simulink model "TargetStatePlant"  (R2019b)
settings: Solver=VariableStepAuto  StartTime=0.0  StopTime=10.0  RelTol=1e-3
undefined symbols (not defined in the file or in its folder): errorMinSpd, heightCalibrating_e, heightDown_e, heightError_e, heightMovingDown_e, heightMovingUp_e, heightUnknown_e, heightUp_e, IOD_OK, IOD_Open, IOD_ScGnd, maxMedianWheelAngle, maxTransitionMachineSpd, minTransitionMachineSpd, trackWidthMax, trackWidthMin, trackWidthTolerance, twoWheelSteer
settings Model: Creator=lemaya  LastModifiedBy=lemaya

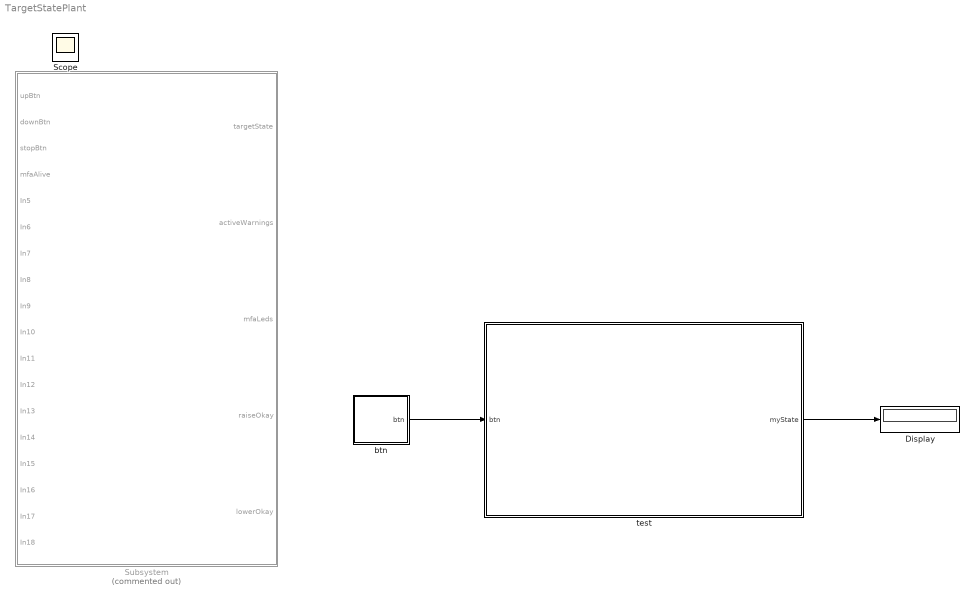
== system TargetStatePlant ==
  Display : Display
  Subsystem : Subsystem  Commented=on
  btn : Stateflow chart  BlockKeywords=__PRM__SERIALIZED__DATA__:Stateflow Chart,Stateflow Diagram  TreatAsAtomicUnit=on
  test : Stateflow chart  BlockKeywords=__PRM__SERIALIZED__DATA__:Stateflow Chart,Stateflow Diagram  TreatAsAtomicUnit=on
  Scope : Scope
  wires:
  test/1(myState) -> Display/1
  btn/1(btn) -> test/1(btn)

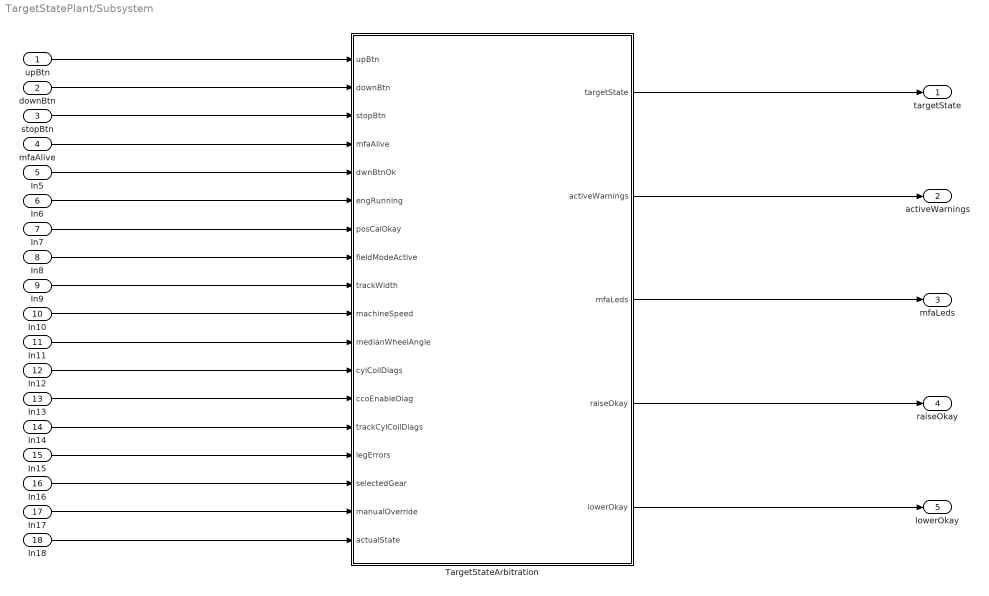
== system TargetStatePlant/Subsystem ==
  upBtn : Inport
  downBtn : Inport  Port=2
  stopBtn : Inport  Port=3
  mfaAlive : Inport  Port=4
  In5 : Inport  Port=5
  In6 : Inport  Port=6
  In7 : Inport  Port=7
  In8 : Inport  Port=8
  In9 : Inport  Port=9
  In10 : Inport  Port=10
  In11 : Inport  Port=11
  In12 : Inport  Port=12
  In13 : Inport  Port=13
  In14 : Inport  Port=14
  In15 : Inport  Port=15
  In16 : Inport  Port=16
  In17 : Inport  Port=17
  In18 : Inport  Port=18
  TargetStateArbitration : Stateflow chart  TreatAsAtomicUnit=on
  targetState : Outport
  activeWarnings : Outport  Port=2
  mfaLeds : Outport  Port=3
  raiseOkay : Outport  Port=4
  lowerOkay : Outport  Port=5
  wires:
  TargetStateArbitration/2(activeWarnings) -> activeWarnings/1
  In8/1 -> TargetStateArbitration/8(fieldModeActive)
  In5/1 -> TargetStateArbitration/5(dwnBtnOk)
  TargetStateArbitration/5(lowerOkay) -> lowerOkay/1
  In16/1 -> TargetStateArbitration/16(selectedGear)
  In18/1 -> TargetStateArbitration/18(actualState)
  TargetStateArbitration/4(raiseOkay) -> raiseOkay/1
  In17/1 -> TargetStateArbitration/17(manualOverride)
  upBtn/1 -> TargetStateArbitration/1(upBtn)
  downBtn/1 -> TargetStateArbitration/2(downBtn)
  In7/1 -> TargetStateArbitration/7(posCalOkay)
  In15/1 -> TargetStateArbitration/15(legErrors)
  TargetStateArbitration/1(targetState) -> targetState/1
  In14/1 -> TargetStateArbitration/14(trackCylCoilDiags)
  In6/1 -> TargetStateArbitration/6(engRunning)
  In11/1 -> TargetStateArbitration/11(medianWheelAngle)
  In12/1 -> TargetStateArbitration/12(cylCoilDiags)
  In13/1 -> TargetStateArbitration/13(ccoEnableDiag)
  In9/1 -> TargetStateArbitration/9(trackWidth)
  In10/1 -> TargetStateArbitration/10(machineSpeed)
  TargetStateArbitration/3(mfaLeds) -> mfaLeds/1
  stopBtn/1 -> TargetStateArbitration/3(stopBtn)
  mfaAlive/1 -> TargetStateArbitration/4(mfaAlive)

== stateflow chart TargetStatePlant/btn ==
  state Off
    en: btn = 0;
  state On
    en: btn = 1;
  (default) -> Off
  Off -> On : after(2,sec)
  On -> Off : after(1,sec)
  data: btn output boolean

== stateflow chart TargetStatePlant/test ==
  state state1
    en: myState = 1;
  state state2
    en: myState = 2;
  state b = leaveState [function]
    (default) -> (junction 8)
    (junction 8) -> (junction 11) [order 1] : [hasChangedTo(btn,1)]
    (junction 11) -> (junction 12) : [myState == 1]
    (junction 8) -> (junction 17) [order 2]
    (junction 12) -> (junction 15) : {b = 1}
    (junction 17) -> (junction 15) : {b = 0}
  (default) -> state1
  state1 -> state2 : [leaveState()]
  state2 -> state1 : [leaveState()]
  data: b function_output double; myState output uint8; btn input boolean

== stateflow chart TargetStatePlant/Subsystem/TargetStateArbitration ==
  state states
    en,du: lowerOkay = ( okayToLower() && !disableLower() );
    raiseOkay = ( okayToRaise() && !disableRiase() );
    state b = leaveActiveState [function]
      (default) -> (junction 1676)
      (junction 1676) -> (junction 1685) [order 1] : [hasChangedTo(stopBtn,1)]
      (junction 1685) -> (junction 1686) [order 1] : [prevTargetState == heightDown_e]
      (junction 1676) -> (junction 1696) [order 2]
      (junction 1685) -> (junction 1687) [order 2]
      (junction 1686) -> (junction 1690)
      (junction 1687) -> (junction 1690) : [prevTargetState == heightUp_e]
      (junction 1690) -> (junction 1698)
      (junction 1696) -> (junction 1698) [order 1] : [manualOverride != 0]
      (junction 1696) -> (junction 1701) [order 2]
      (junction 1698) -> (junction 1700)
      (junction 1701) -> (junction 1700) [order 1] : [!calOkay()]
      (junction 1701) -> (junction 1711) [order 2]
      (junction 1700) -> (junction 1712)
      (junction 1711) -> (junction 1705) [order 1] : [prevTargetState == heightMovingDown_e]
      (junction 1705) -> (junction 1712) : [disableLower()]
      (junction 1711) -> (junction 1713) [order 2]
      (junction 1712) -> (junction 1714)
      (junction 1713) -> (junction 1706) [order 1] : [prevTargetState == heightMovingUp_e]
      (junction 1706) -> (junction 1714) : [disableRiase()]
      (junction 1713) -> (junction 1716) [order 2]
      (junction 1714) -> (junction 1717)
      (junction 1716) -> (junction 1717) [order 1] : [noMovementErr()]
      (junction 1716) -> (junction 1742) [order 2]
      (junction 1717) -> (junction 1734)
      (junction 1742) -> (junction 1733) [order 2] : [hasChangedTo(downBtn,1)]
      (junction 1733) -> (junction 1734) : [prevTargetState == heightMovingDown_e]
      (junction 1742) -> (junction 1744) [order 1]
      (junction 1734) -> (junction 1738)
      (junction 1744) -> (junction 1737) [order 1] : [hasChangedTo(downBtn,1)]
      (junction 1737) -> (junction 1738) : [prevTargetState == heightMovingUp_e]
      (junction 1744) -> (junction 1725) [order 2]
      (junction 1738) -> (junction 1728)
      (junction 1728) -> (junction 1730) : {b = true}
      (junction 1730) -> (junction 1723)
      (junction 1725) -> (junction 1723) : {b = false}
    state clearWarnings [function]
      (default) -> (junction 687) : {activeWarnings.trackWidth = 0;
          | activeWarnings.speed = 0;
          | activeWarnings.guide = 0;
          | activeWarnings.was = 0;
          | activeWarnings.fws = 0;
          | activeWarnings.fieldRoad = 0;
          | activeWarnings.cal = 0;
          | activeWarnings.parkBrake = 0;}
    state upWarnings [function]
      (default) -> (junction 973) : {activeWarnings.trackWidth = !trackWidthOkay();
          | activeWarnings.speed = !speedOkay();
          | activeWarnings.guide = 0;
          | activeWarnings.was = !wasOkay();
          | activeWarnings.fws = 0;
          | activeWarnings.fieldRoad = !fieldModeActive;
          | activeWarnings.cal = !calOkay();
          | activeWarnings.parkBrake = 0;}
    state downWarnings [function]
      (default) -> (junction 976) : {activeWarnings.trackWidth = !trackWidthOkay();
          | activeWarnings.speed = !speedOkay();
          | activeWarnings.guide = 0;
          | activeWarnings.was = !wasOkay();
          | activeWarnings.fws = 0;
          | activeWarnings.fieldRoad = !fieldModeActive;
          | activeWarnings.cal = !calOkay();
          | activeWarnings.parkBrake = !parkBrakeOkay();}
    state doNothing
      en:
      targetState = heightUnknown_e;
      clearWarnings();
      mfaLeds.downBtn = 0;
      mfaLeds.upBtn = 0;
    state active
      en: clearWarnings();
      (history)
      state paused
        en:
        targetState = heightUnknown_e;
      state wait
        en:
        clearWarnings();
      state out = pauseTransition [function]
        (default) -> (junction 927)
        (junction 927) -> (junction 981) [order 1] : [targetState == heightMovingUp_e]
        (junction 981) -> (junction 931) : [!okayToRaise()]
        (junction 931) -> (junction 984) : {upWarnings()}
        (junction 927) -> (junction 933) [order 2]
        (junction 984) -> (junction 937)
        (junction 986) -> (junction 988) : [!okayToLower()]
        (junction 988) -> (junction 937) : {downWarnings()}
        (junction 933) -> (junction 986) [order 1] : [targetState == heightMovingDown_e]
        (junction 933) -> (junction 991) [order 2]
        (junction 937) -> (junction 938) : {out = true}
        (junction 991) -> (junction 932)
        (junction 932) -> (junction 938) : {out = false}
      state out = restartTransition [function]
        (default) -> (junction 1027)
        (junction 1027) -> (junction 1028) [order 1] : [prevTargetState == heightMovingUp_e]
        (junction 1028) -> (junction 1029) : [okayToRaise()]
        (junction 1027) -> (junction 1030) [order 2]
        (junction 1029) -> (junction 1032)
        (junction 1030) -> (junction 1031) [order 1] : [prevTargetState == heightMovingDown_e]
        (junction 1031) -> (junction 1032) : [okayToLower()]
        (junction 1030) -> (junction 1034) [order 2]
        (junction 1032) -> (junction 1035) : {out = true}
        (junction 1034) -> (junction 1035) : {out = false}
      state transitioning
        (history)
        state up
          en:
          targetState = heightMovingUp_e;
          prevTargetState = heightMovingUp_e;
          mfaLeds.upBtn = 2;
          mfaLeds.downBtn = 0;
        state down
          en:
          targetState = heightMovingDown_e;
          prevTargetState = heightMovingDown_e;
          mfaLeds.upBtn = 0;
          mfaLeds.downBtn = 2;
      state holdUp
        en:
        targetState = heightUp_e;
        prevTargetState = heightUp_e;
        mfaLeds.upBtn = 1;
        mfaLeds.downBtn = 0;
      state holdDown
        en:
        targetState = heightDown_e;
        prevTargetState = heightDown_e;
        mfaLeds.upBtn = 0;
        mfaLeds.downBtn = 1;
      paused -> wait : after(20,msec)
      transitioning -> paused : [pauseTransition()]
      wait -> (junction 1563) : [restartTransition()]
      (junction 1563) -> transitioning
      up -> holdUp : [actualState == heightUp_e]
      down -> holdDown : [actualState == heightDown_e]
    state updateWarningsUp
      en: upWarnings();
    state updateWarningsDown
      en: downWarnings();
    state waitForEngineRunning
      en:
      targetState = heightUnknown_e;
      mfaLeds.downBtn = 0;
      mfaLeds.upBtn = 0;
    state out = okayToLower [function]
      (junction 1653) -> (junction 1652) : [trackWidthOkay()]
      (junction 741) -> (junction 1653) [order 2]
      (junction 1652) -> (junction 742)
      (default) -> (junction 737)
      (junction 739) -> (junction 740)
      (junction 737) -> (junction 1545) [order 1] : [parkBrakeOkay()]
      (junction 1545) -> (junction 738) : [speedOkay()]
      (junction 738) -> (junction 739) : [wasOkay()]
      (junction 740) -> (junction 741) : [fieldModeActive]
      (junction 741) -> (junction 742) [order 1] : [trackWidthError()]
      (junction 737) -> (junction 743) [order 2]
      (junction 742) -> (junction 748) : {out = true}
      (junction 743) -> (junction 748) : {out = false}
    state out = disableLower [function]
      (default) -> (junction 1251)
      (junction 1251) -> (junction 1400) [order 1] : [prevTargetState == heightMovingDown_e]
      (junction 1400) -> (junction 1252) : [!mfaAlive]
      (junction 1251) -> (junction 1415) [order 2]
      (junction 1252) -> (junction 1407)
      (junction 1415) -> (junction 1265)
      (junction 1407) -> (junction 1266) : {out = true}
      (junction 1265) -> (junction 1266) : {out = false}
    state out = trackWidthError [function]
      (default) -> (junction 834)
      (junction 834) -> (junction 835) [order 1] : [trackWidth.FrontLeft <= 0]
      (junction 834) -> (junction 836) [order 2]
      (junction 835) -> (junction 837)
      (junction 836) -> (junction 837) [order 1] : [trackWidth.FrontRight <= 0]
      (junction 836) -> (junction 838) [order 2]
      (junction 837) -> (junction 839)
      (junction 838) -> (junction 839) [order 1] : [trackWidth.RearLeft <= 0]
      (junction 838) -> (junction 840) [order 2]
      (junction 839) -> (junction 841)
      (junction 840) -> (junction 841) [order 1] : [trackWidth.RearRight <= 0]
      (junction 840) -> (junction 842) [order 2] : {out = false}
      (junction 841) -> (junction 843) : {out = true}
      (junction 843) -> (junction 842)
    state out = trackRngCheck(width) [function]
      (default) -> (junction 782)
      (junction 782) -> (junction 783) [order 1] : [!trackWidthError()]
      (junction 783) -> (junction 784) : [width >= (trackWidthMin - trackWidthTolerance)]
      (junction 782) -> (junction 785) [order 2] : {out = false}
      (junction 784) -> (junction 786) : [width <= (trackWidthMax + trackWidthTolerance)]
      (junction 786) -> (junction 785) : {out = true}
    state out = requireSpeed [function]
      (default) -> (junction 718)
      (junction 718) -> (junction 719) [commented out] : [trackWidthError()]
      (junction 719) -> (junction 721) [commented out]
      (junction 718) -> (junction 720)
      (junction 720) -> (junction 721) [commented out] : [actualState == heightError_e]
      (junction 720) -> (junction 1581)
      (junction 721) -> (junction 1579) [commented out]
      (junction 1581) -> (junction 1579) [commented out] : [!calOkay()]
      (junction 1581) -> (junction 1107)
      (junction 1579) -> (junction 1109) [commented out]
      (junction 1107) -> (junction 1109) [commented out] : [(cylCoilDiags.retract.FrontLeft & IOD_Open) == IOD_Open]
      (junction 1107) -> (junction 1113)
      (junction 1109) -> (junction 1114) [commented out]
      (junction 1113) -> (junction 1114) [commented out] : [(cylCoilDiags.retract.FrontRight & IOD_Open) == IOD_Open]
      (junction 1114) -> (junction 1122) [commented out]
      (junction 1113) -> (junction 1121)
      (junction 1121) -> (junction 1122) [commented out] : [(cylCoilDiags.retract.RearLeft & IOD_Open) == IOD_Open]
      (junction 1122) -> (junction 1125) [commented out]
      (junction 1121) -> (junction 1124)
      (junction 1124) -> (junction 1125) [commented out] : [(cylCoilDiags.retract.RearRight & IOD_Open) == IOD_Open]
      (junction 1125) -> (junction 722) [commented out]
      (junction 1124) -> (junction 1180)
      (junction 1180) -> (junction 722) [commented out] : [trackCylError()]
      (junction 1180) -> (junction 723)
      (junction 722) -> (junction 724) [commented out] : {out = true}
      (junction 723) -> (junction 724) : {out = false}
    state out = calOkay [function]
      (default) -> (junction 768)
      (junction 768) -> (junction 769) [order 1] : [actualState != heightCalibrating_e]
      (junction 768) -> (junction 771) [order 2] : {out = false}
      (junction 769) -> (junction 770) : [posCalOkay]
      (junction 770) -> (junction 772) : {out = true}
      (junction 771) -> (junction 772)
    state out = wasOkay [function]
      note: %No Front wheel angle requirement
      (default) -> (junction 795)
      (junction 795) -> (junction 1667) [order 1] : [1==1]
      (junction 795) -> (junction 1663) [order 2] : [abs(medianWheelAngle) > maxMedianWheelAngle]
      (junction 1667) -> (junction 1668)
      (junction 795) -> (junction 1665) [order 3] : [!prevWasOkayOut]
      (junction 1663) -> (junction 798) : {out = false}
      (junction 1665) -> (junction 796) : [abs(medianWheelAngle) <= (maxMedianWheelAngle - 2)]
      (junction 1668) -> (junction 796)
      (junction 796) -> (junction 798) : {out = true}
      (junction 798) -> (junction 1660) : {prevWasOkayOut = out}
    state out = targetStateSelected [function]
      (default) -> (junction 1068)
      (junction 1068) -> (junction 1069) [order 1] : [targetState == heightDown_e]
      (junction 1068) -> (junction 1070) [order 2]
      (junction 1069) -> (junction 1071)
      (junction 1070) -> (junction 1071) [order 1] : [targetState == heightUp_e]
      (junction 1070) -> (junction 1085) [order 2]
      (junction 1071) -> (junction 1091)
      (junction 1085) -> (junction 1091) [order 1] : [targetState == heightMovingUp_e]
      (junction 1085) -> (junction 1092) [order 2]
      (junction 1091) -> (junction 1087)
      (junction 1092) -> (junction 1087) [order 1] : [targetState == heightMovingDown_e]
      (junction 1092) -> (junction 1073) [order 2]
      (junction 1087) -> (junction 1074) : {out = true}
      (junction 1073) -> (junction 1074) : {out = false}
    state out = okayToRaise [function]
      (default) -> (junction 894)
      (junction 1304) -> (junction 1298)
      (junction 894) -> (junction 1547) [order 1]
      (junction 1547) -> (junction 1247)
      (junction 1247) -> (junction 1195) : [trackWidthOkay()]
      (junction 1195) -> (junction 1305) : [speedOkay()]
      (junction 1305) -> (junction 1304) : [wasOkay()]
      (junction 1298) -> (junction 896) : [fieldModeActive]
      (junction 894) -> (junction 897) [order 2]
      (junction 896) -> (junction 899) : {out = true}
      (junction 897) -> (junction 899) : {out = false}
    state out = disableRiase [function]
      (default) -> (junction 1420)
      (junction 1420) -> (junction 1448) [order 1] : [prevTargetState == heightMovingUp_e]
      (junction 1448) -> (junction 1635) [order 1] : [!mfaAlive]
      (junction 1420) -> (junction 1423) [order 2]
      (junction 1448) -> (junction 1421) [order 2]
      (junction 1635) -> (junction 1422)
      (junction 1423) -> (junction 1421) [order 1] : [prevTargetState == heightDown_e]
      (junction 1421) -> (junction 1422) [order 1] : [trackWidthError()]
      (junction 1423) -> (junction 1426) [order 2]
      (junction 1421) -> (junction 1424) [order 2]
      (junction 1422) -> (junction 1425)
      (junction 1424) -> (junction 1425) [order 1] : [trackCylError()]
      (junction 1424) -> (junction 1647) [order 2]
      (junction 1425) -> (junction 1650)
      (junction 1647) -> (junction 1650) [order 1] : [!dwnBtnOk]
      (junction 1647) -> (junction 1457) [order 2]
      (junction 1650) -> (junction 1446)
      (junction 1457) -> (junction 1446) [order 1] : [actualState == heightError_e]
      (junction 1457) -> (junction 1464) [order 2]
      (junction 1446) -> (junction 1466)
      (junction 1464) -> (junction 1466) [order 1] : [cylCoilDiags.extend.FrontLeft != IOD_OK]
      (junction 1464) -> (junction 1470) [order 2]
      (junction 1466) -> (junction 1468)
      (junction 1470) -> (junction 1468) [order 1] : [cylCoilDiags.extend.FrontRight != IOD_OK]
      (junction 1470) -> (junction 1473) [order 2]
      (junction 1468) -> (junction 1471)
      (junction 1473) -> (junction 1471) [order 1] : [cylCoilDiags.extend.RearLeft != IOD_OK]
      (junction 1473) -> (junction 1476) [order 2]
      (junction 1471) -> (junction 1474)
      (junction 1476) -> (junction 1474) [order 1] : [cylCoilDiags.extend.RearRight != IOD_OK]
      (junction 1476) -> (junction 1495) [order 2]
      (junction 1474) -> (junction 1485)
      (junction 1495) -> (junction 1485) [order 1] : [cylCoilDiags.retract.FrontLeft != IOD_OK]
      (junction 1495) -> (junction 1489) [order 2]
      (junction 1485) -> (junction 1487)
      (junction 1489) -> (junction 1487) [order 1] : [cylCoilDiags.retract.FrontRight != IOD_OK]
      (junction 1489) -> (junction 1488) [order 2]
      (junction 1487) -> (junction 1484)
      (junction 1488) -> (junction 1484) [order 1] : [cylCoilDiags.retract.RearLeft != IOD_OK]
      (junction 1488) -> (junction 1498) [order 2]
      (junction 1484) -> (junction 1493)
      (junction 1498) -> (junction 1493) [order 1] : [cylCoilDiags.retract.RearRight != IOD_OK]
      (junction 1498) -> (junction 1452) [order 2]
      (junction 1493) -> (junction 1427) : {out = true}
      (junction 1426) -> (junction 1452)
      (junction 1452) -> (junction 1427) : {out = false}
    state out = trackCylError [function]
      (default) -> (junction 1136)
      (junction 1136) -> (junction 1137) [order 1] : [trackCylCoilDiags.extend.FrontLeft != IOD_OK]
      (junction 1136) -> (junction 1138) [order 2]
      (junction 1137) -> (junction 1139)
      (junction 1138) -> (junction 1139) [order 1] : [trackCylCoilDiags.extend.FrontRight != IOD_OK]
      (junction 1138) -> (junction 1140) [order 2]
      (junction 1139) -> (junction 1141)
      (junction 1140) -> (junction 1141) [order 1] : [trackCylCoilDiags.extend.RearLeft != IOD_OK]
      (junction 1140) -> (junction 1142) [order 2]
      (junction 1141) -> (junction 1143)
      (junction 1142) -> (junction 1143) [order 1] : [trackCylCoilDiags.extend.RearRight != IOD_OK]
      (junction 1142) -> (junction 1163) [order 2]
      (junction 1143) -> (junction 1167)
      (junction 1163) -> (junction 1167) [order 1] : [trackCylCoilDiags.retract.FrontLeft != IOD_OK]
      (junction 1163) -> (junction 1161) [order 2]
      (junction 1167) -> (junction 1160)
      (junction 1161) -> (junction 1160) [order 1] : [trackCylCoilDiags.retract.FrontRight != IOD_OK]
      (junction 1161) -> (junction 1162) [order 2]
      (junction 1160) -> (junction 1170)
      (junction 1162) -> (junction 1170) [order 1] : [trackCylCoilDiags.retract.RearLeft != IOD_OK]
      (junction 1162) -> (junction 1174) [order 2]
      (junction 1170) -> (junction 1173)
      (junction 1174) -> (junction 1173) [order 1] : [trackCylCoilDiags.retract.RearRight != IOD_OK]
      (junction 1174) -> (junction 1144) [order 2] : {out = false}
      (junction 1173) -> (junction 1145) : {out = true}
      (junction 1145) -> (junction 1144)
    state out = trackWidthOkay [function]
      (default) -> (junction 807)
      (junction 807) -> (junction 806) [order 2]
      (junction 806) -> (junction 808)
      (junction 807) -> (junction 809) [order 1] : [trackRngCheck(trackWidth.FrontLeft)]
      (junction 809) -> (junction 808) [order 2]
      (junction 808) -> (junction 810)
      (junction 809) -> (junction 811) [order 1] : [trackRngCheck(trackWidth.FrontRight)]
      (junction 811) -> (junction 810) [order 2]
      (junction 810) -> (junction 812)
      (junction 811) -> (junction 813) [order 1] : [trackRngCheck(trackWidth.RearLeft)]
      (junction 813) -> (junction 812) [order 2]
      (junction 812) -> (junction 815) : {out = false}
      (junction 813) -> (junction 814) [order 1] : [trackRngCheck(trackWidth.RearRight)]
      (junction 814) -> (junction 816) : {out = true}
      (junction 815) -> (junction 816)
    state out = speedOkay [function]
      (default) -> (junction 871)
      (junction 871) -> (junction 872) [order 1] : [requireSpeed()]
      (junction 872) -> (junction 873) : [machineSpeed > errorMinSpd]
      (junction 871) -> (junction 874) [order 2]
      (junction 873) -> (junction 875)
      (junction 874) -> (junction 875) [order 1] : [machineSpeed >= minTransitionMachineSpd]
      (junction 875) -> (junction 876) [order 1] : [machineSpeed <= maxTransitionMachineSpd]
      (junction 874) -> (junction 879) [order 2]
      (junction 875) -> (junction 877) [order 2]
      (junction 876) -> (junction 878) : {out = true}
      (junction 877) -> (junction 878) : {out = false}
      (junction 879) -> (junction 877)
    state out = targetStateDown [function]
      (default) -> (junction 1320)
      (junction 1320) -> (junction 1321) [order 1] : [targetState == heightDown_e]
      (junction 1320) -> (junction 1322) [order 2]
      (junction 1321) -> (junction 1323)
      (junction 1322) -> (junction 1323) [order 1] : [targetState == heightMovingDown_e]
      (junction 1322) -> (junction 1334) [order 2]
      (junction 1323) -> (junction 1335) : {out = true}
      (junction 1334) -> (junction 1335) : {out = false}
    state out = targetStateUp [function]
      (default) -> (junction 1361)
      (junction 1361) -> (junction 1362) [order 1] : [targetState == heightUp_e]
      (junction 1361) -> (junction 1363) [order 2]
      (junction 1362) -> (junction 1364)
      (junction 1363) -> (junction 1364) [order 1] : [targetState == heightMovingUp_e]
      (junction 1363) -> (junction 1375) [order 2]
      (junction 1364) -> (junction 1376) : {out = true}
      (junction 1375) -> (junction 1376) : {out = false}
    state out = noMovementErr [function]
      (default) -> (junction 1516)
      (junction 1516) -> (junction 1518) [order 1] : [legErrors.FrontLeft.noMovementErr]
      (junction 1516) -> (junction 1515) [order 2]
      (junction 1518) -> (junction 1520)
      (junction 1515) -> (junction 1520) [order 1] : [legErrors.FrontRight.noMovementErr]
      (junction 1515) -> (junction 1517) [order 2]
      (junction 1520) -> (junction 1522)
      (junction 1517) -> (junction 1522) [order 1] : [legErrors.RearLeft.noMovementErr]
      (junction 1517) -> (junction 1519) [order 2]
      (junction 1522) -> (junction 1523)
      (junction 1519) -> (junction 1523) [order 1] : [legErrors.RearRight.noMovementErr]
      (junction 1519) -> (junction 1524) [order 2] : {out = false}
      (junction 1523) -> (junction 1525) : {out = true}
      (junction 1524) -> (junction 1525)
    state out = parkBrakeOkay [function]
      (default) -> (junction 1551)
      (junction 1551) -> (junction 1552) [order 1] : [selectedGear != 251]
      (junction 1551) -> (junction 1553) [order 2] : {out = false}
      (junction 1552) -> (junction 1554) : {out = true}
      (junction 1554) -> (junction 1553)
    active -> doNothing [order 1] : [leaveActiveState()]
    (junction 705) -> doNothing [order 2]
    (junction 705) -> active [order 1] : [targetStateSelected()]
    updateWarningsUp -> (junction 705) : after(20,msec)
    (junction 1628) -> up : [!disableRiase()]
    (junction 1624) -> (junction 1628) [order 2] : [okayToRaise()]
    (junction 1569) -> holdUp
    (junction 1567) -> (junction 1569)
    (junction 267) -> updateWarningsUp [order 2]
    doNothing -> (junction 267) [order 1] : [hasChangedTo(upBtn,1)]
    (junction 267) -> (junction 1624) [order 1] : [calOkay()]
    (junction 1624) -> holdUp [order 1] : [actualState == heightUp_e]
    (junction 270) -> (junction 267)
    (junction 1197) -> (junction 270) : [targetStateDown()]
    active -> (junction 1197) [order 2] : [hasChangedTo(upBtn,1)]
    (junction 1199) -> (junction 282) : [targetStateUp()]
    active -> (junction 1199) [order 3] : [hasChangedTo(downBtn,1)]
    (junction 282) -> (junction 125)
    doNothing -> (junction 125) [order 2] : [hasChangedTo(downBtn,1)]
    (junction 125) -> (junction 1619) [order 1] : [calOkay()]
    (junction 1619) -> holdDown [order 1] : [actualState == heightDown_e]
    (junction 125) -> updateWarningsDown [order 2]
    (junction 1619) -> (junction 1630) [order 2] : [okayToLower() ]
    (junction 1630) -> down : [!disableLower()]
    updateWarningsDown -> (junction 702) : after(20,msec)
    (junction 1566) -> holdDown [order 1] : [actualState == heightDown_e]
    (junction 702) -> doNothing [order 2]
    (junction 702) -> active [order 1] : [targetStateSelected()]
    (junction 1575) -> doNothing
    (junction 1613) -> (junction 1575)
    (junction 1616) -> (junction 1613)
    (junction 1566) -> (junction 1616) [order 2]
    (junction 1609) -> (junction 1613) [order 2]
    (junction 1611) -> (junction 1616) [order 2]
    (junction 1572) -> (junction 1566) [order 2]
    waitForEngineRunning -> (junction 1609) : [engRunning]
    (junction 1609) -> (junction 1611) [order 1] : [fieldModeActive]
    (junction 1611) -> (junction 1572) [order 1] : [calOkay()]
    (junction 1572) -> (junction 1567) [order 1] : [actualState == heightUp_e]
    (default) -> waitForEngineRunning
  (default) -> states
  states -> states : [hasChangedTo(engRunning,0)]
  data: b function_output double; out function_output double; out function_output double; out function_output boolean; out function_output boolean; out function_output boolean; out function_output boolean; width function_input single; out function_output boolean; out function_output boolean; out function_output boolean; out function_output boolean; out function_output boolean; out function_output boolean; out function_output boolean; out function_output boolean; out function_output boolean; out function_output boolean; out function_output boolean; out function_output boolean; out function_output boolean; heightDown_e parameter; heightUp_e parameter; heightCalibrating_e parameter; heightError_e parameter; heightUnknown_e parameter; upBtn input; downBtn input; stopBtn input; mfaAlive input boolean; dwnBtnOk input boolean; targetState output uint8; twoWheelSteer parameter; maxMedianWheelAngle parameter; maxTransitionMachineSpd parameter; minTransitionMachineSpd parameter; activeWarnings output Bus: UserWarningBus; mfaLeds output Bus: MfaBus =0; trackWidthMin parameter; trackWidthMax parameter; engRunning input boolean; posCalOkay input; fieldModeActive input boolean; trackWidth input Bus: CylinderBus; machineSpeed input; medianWheelAngle input; cylCoilDiags input Bus: CoilStateBus; ccoEnableDiag input; trackCylCoilDiags input Bus: CoilStateBus; legErrors input Bus: ErrorsBus; selectedGear input; manualOverride input; actualState input; errorMinSpd parameter; prevTargetState local uint8; heightMovingDown_e parameter; heightMovingUp_e parameter; raiseOkay output boolean; lowerOkay output boolean; IOD_Open parameter; IOD_ScGnd parameter; IOD_OK parameter; prevWasOkayOut local boolean =0; trackWidthTolerance parameter
